simulink model "PWM_Generator"  (R2014a)
settings: Solver=ode45  StartTime=0.0  StopTime=50000  RelTol=1e-3
libraries: hdlsllib x20, simulink x5
settings Model: Creator=diloreto.m  LastModifiedBy=diloreto.m

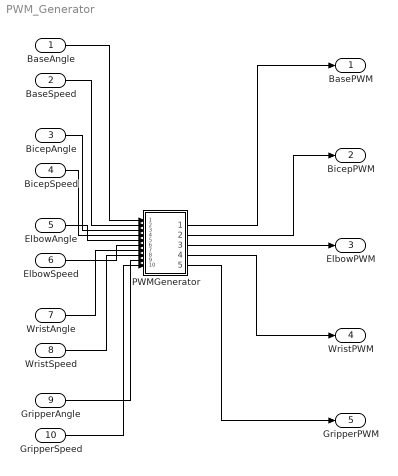
== system PWM_Generator ==
  BaseAngle : Inport  OutDataTypeStr=uint8  SampleTime=1
  BaseSpeed : Inport  Port=2  OutDataTypeStr=uint8  SampleTime=1
  BicepAngle : Inport  Port=3  OutDataTypeStr=uint8  SampleTime=1
  BicepSpeed : Inport  Port=4  OutDataTypeStr=uint8  SampleTime=1
  ElbowAngle : Inport  Port=5  OutDataTypeStr=uint8  SampleTime=1
  ElbowSpeed : Inport  Port=6  OutDataTypeStr=uint8  SampleTime=1
  WristAngle : Inport  Port=7  OutDataTypeStr=uint8  SampleTime=1
  WristSpeed : Inport  Port=8  OutDataTypeStr=uint8  SampleTime=1
  GripperAngle : Inport  Port=9  OutDataTypeStr=uint8  SampleTime=1
  GripperSpeed : Inport  Port=10  OutDataTypeStr=uint8  SampleTime=1
  PWMGenerator : Subsystem  TreatAsAtomicUnit=on  SystemSampleTime=1
  BasePWM : Outport
  BicepPWM : Outport  Port=2
  ElbowPWM : Outport  Port=3
  WristPWM : Outport  Port=4
  GripperPWM : Outport  Port=5
  wires:
  BaseAngle/1 -> PWMGenerator/1(BaseAngle)
  BaseSpeed/1 -> PWMGenerator/2(BaseSpeed)
  BicepAngle/1 -> PWMGenerator/3(BicepAngle)
  BicepSpeed/1 -> PWMGenerator/4(BicepSpeed)
  ElbowAngle/1 -> PWMGenerator/5(ElbowAngle)
  ElbowSpeed/1 -> PWMGenerator/6(ElbowSpeed)
  WristAngle/1 -> PWMGenerator/7(WristAngle)
  WristSpeed/1 -> PWMGenerator/8(WristSpeed)
  GripperAngle/1 -> PWMGenerator/9(GripperAngle)
  GripperSpeed/1 -> PWMGenerator/10(GripperSpeed)
  PWMGenerator/1(BasePWM) -> BasePWM/1
  PWMGenerator/2(BicepPWM) -> BicepPWM/1
  PWMGenerator/3(ElbowPWM) -> ElbowPWM/1
  PWMGenerator/4(WristPWM) -> WristPWM/1
  PWMGenerator/5(GripperPWM) -> GripperPWM/1

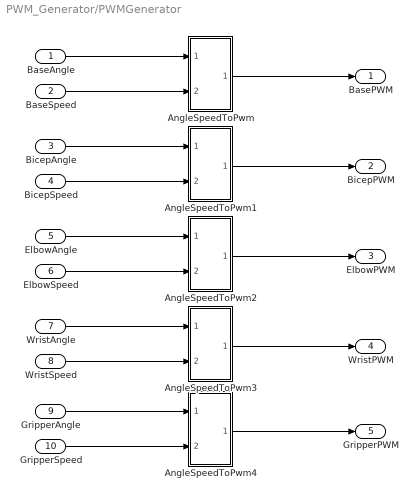
== system PWM_Generator/PWMGenerator ==
  BaseAngle : Inport  OutDataTypeStr=uint8  SampleTime=1
  BaseSpeed : Inport  Port=2  OutDataTypeStr=uint8  SampleTime=1
  BicepAngle : Inport  Port=3  OutDataTypeStr=uint8  SampleTime=1
  BicepSpeed : Inport  Port=4  OutDataTypeStr=uint8  SampleTime=1
  ElbowAngle : Inport  Port=5  OutDataTypeStr=uint8  SampleTime=1
  ElbowSpeed : Inport  Port=6  OutDataTypeStr=uint8  SampleTime=1
  WristAngle : Inport  Port=7  OutDataTypeStr=uint8  SampleTime=1
  WristSpeed : Inport  Port=8  OutDataTypeStr=uint8  SampleTime=1
  GripperAngle : Inport  Port=9  OutDataTypeStr=uint8  SampleTime=1
  GripperSpeed : Inport  Port=10  OutDataTypeStr=uint8  SampleTime=1
  AngleSpeedToPwm : Subsystem
  AngleSpeedToPwm1 : Subsystem
  AngleSpeedToPwm2 : Subsystem
  AngleSpeedToPwm3 : Subsystem
  AngleSpeedToPwm4 : Subsystem
  BasePWM : Outport
  BicepPWM : Outport  Port=2
  ElbowPWM : Outport  Port=3
  WristPWM : Outport  Port=4
  GripperPWM : Outport  Port=5
  wires:
  AngleSpeedToPwm2/1(PWM) -> ElbowPWM/1
  ElbowSpeed/1 -> AngleSpeedToPwm2/2(Speed)
  ElbowAngle/1 -> AngleSpeedToPwm2/1(Angle)
  WristAngle/1 -> AngleSpeedToPwm3/1(Angle)
  WristSpeed/1 -> AngleSpeedToPwm3/2(Speed)
  AngleSpeedToPwm3/1(PWM) -> WristPWM/1
  GripperAngle/1 -> AngleSpeedToPwm4/1(Angle)
  GripperSpeed/1 -> AngleSpeedToPwm4/2(Speed)
  AngleSpeedToPwm4/1(PWM) -> GripperPWM/1
  BaseSpeed/1 -> AngleSpeedToPwm/2(Speed)
  BaseAngle/1 -> AngleSpeedToPwm/1(Angle)
  AngleSpeedToPwm/1(PWM) -> BasePWM/1
  AngleSpeedToPwm1/1(PWM) -> BicepPWM/1
  BicepAngle/1 -> AngleSpeedToPwm1/1(Angle)
  BicepSpeed/1 -> AngleSpeedToPwm1/2(Speed)

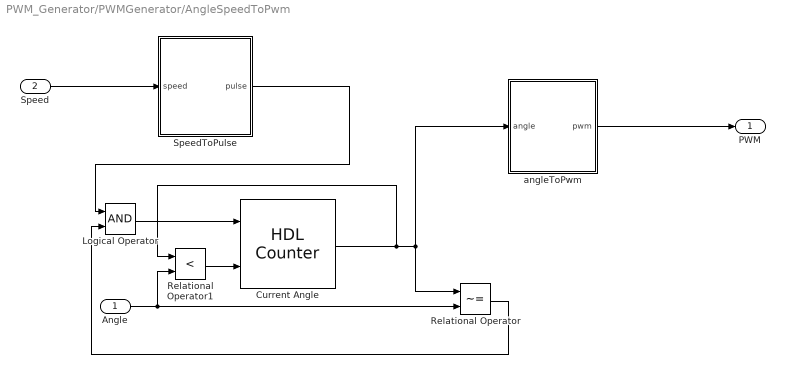
== system PWM_Generator/PWMGenerator/AngleSpeedToPwm ==
  Angle : Inport  OutDataTypeStr=uint8  SampleTime=1
  Speed : Inport  Port=2  OutDataTypeStr=uint8  SampleTime=1
  Current Angle : hdlsllib/HDL Operations/HDL Counter  CountType=Count limited  CountInit=90  CountStep=1  CountMax=180  CountFromType=Specify  CountFrom=0  CountResetPort=off  CountLoadPort=off  CountEnbPort=on  CountDirPort=on  CountDataType=Unsigned  CountWordLen=8  CountFracLen=0  CountSampTime=1
  Logical Operator : Logic  AllPortsSameDT=off  OutDataTypeStr=boolean  SampleTime=1
  Relational Operator : RelationalOperator  Operator=~=  OutDataTypeStr=boolean  SampleTime=1
  Relational Operator1 : RelationalOperator  Operator=<  OutDataTypeStr=boolean  SampleTime=1
  SpeedToPulse : Subsystem
  angleToPwm : Subsystem
  PWM : Outport  OutDataTypeStr=boolean  SampleTime=1
  wires:
  Current Angle/1 -> Relational Operator1/1, Relational Operator/1, angleToPwm/1(angle)
  Relational Operator1/1 -> Current Angle/2
  Angle/1 -> Relational Operator1/2, Relational Operator/2
  angleToPwm/1(pwm) -> PWM/1
  Speed/1 -> SpeedToPulse/1(speed)
  Logical Operator/1 -> Current Angle/1
  Relational Operator/1 -> Logical Operator/2
  SpeedToPulse/1(pulse) -> Logical Operator/1

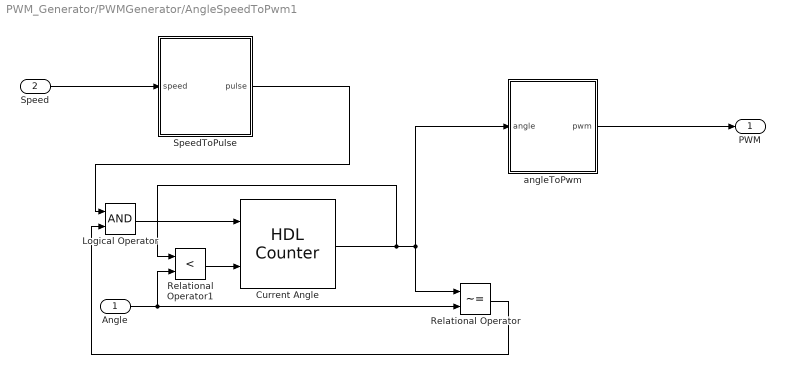
== system PWM_Generator/PWMGenerator/AngleSpeedToPwm1 ==
  Angle : Inport  OutDataTypeStr=uint8  SampleTime=1
  Speed : Inport  Port=2  OutDataTypeStr=uint8  SampleTime=1
  Current Angle : hdlsllib/HDL Operations/HDL Counter  CountType=Count limited  CountInit=90  CountStep=1  CountMax=180  CountFromType=Specify  CountFrom=0  CountResetPort=off  CountLoadPort=off  CountEnbPort=on  CountDirPort=on  CountDataType=Unsigned  CountWordLen=8  CountFracLen=0  CountSampTime=1
  Logical Operator : Logic  AllPortsSameDT=off  OutDataTypeStr=boolean  SampleTime=1
  Relational Operator : RelationalOperator  Operator=~=  OutDataTypeStr=boolean  SampleTime=1
  Relational Operator1 : RelationalOperator  Operator=<  OutDataTypeStr=boolean  SampleTime=1
  SpeedToPulse : Subsystem
  angleToPwm : Subsystem
  PWM : Outport  OutDataTypeStr=boolean  SampleTime=1
  wires:
  Current Angle/1 -> Relational Operator1/1, Relational Operator/1, angleToPwm/1(angle)
  Relational Operator1/1 -> Current Angle/2
  Angle/1 -> Relational Operator1/2, Relational Operator/2
  angleToPwm/1(pwm) -> PWM/1
  Speed/1 -> SpeedToPulse/1(speed)
  Logical Operator/1 -> Current Angle/1
  Relational Operator/1 -> Logical Operator/2
  SpeedToPulse/1(pulse) -> Logical Operator/1

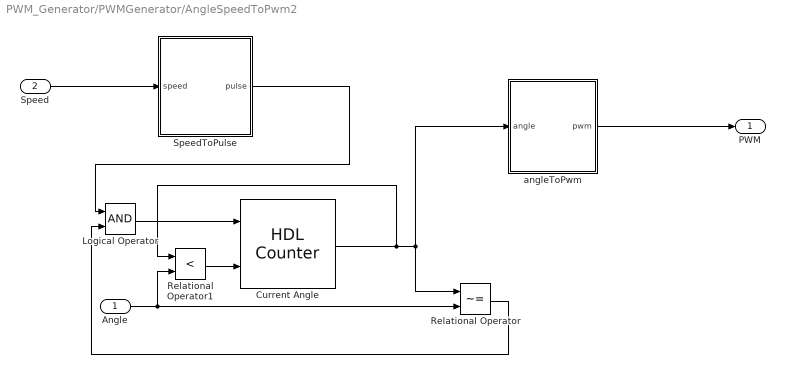
== system PWM_Generator/PWMGenerator/AngleSpeedToPwm2 ==
  Angle : Inport  OutDataTypeStr=uint8  SampleTime=1
  Speed : Inport  Port=2  OutDataTypeStr=uint8  SampleTime=1
  Current Angle : hdlsllib/HDL Operations/HDL Counter  CountType=Count limited  CountInit=90  CountStep=1  CountMax=180  CountFromType=Specify  CountFrom=0  CountResetPort=off  CountLoadPort=off  CountEnbPort=on  CountDirPort=on  CountDataType=Unsigned  CountWordLen=8  CountFracLen=0  CountSampTime=1
  Logical Operator : Logic  AllPortsSameDT=off  OutDataTypeStr=boolean  SampleTime=1
  Relational Operator : RelationalOperator  Operator=~=  OutDataTypeStr=boolean  SampleTime=1
  Relational Operator1 : RelationalOperator  Operator=<  OutDataTypeStr=boolean  SampleTime=1
  SpeedToPulse : Subsystem
  angleToPwm : Subsystem
  PWM : Outport  OutDataTypeStr=boolean  SampleTime=1
  wires:
  Current Angle/1 -> Relational Operator1/1, Relational Operator/1, angleToPwm/1(angle)
  Relational Operator1/1 -> Current Angle/2
  Angle/1 -> Relational Operator1/2, Relational Operator/2
  angleToPwm/1(pwm) -> PWM/1
  Speed/1 -> SpeedToPulse/1(speed)
  Logical Operator/1 -> Current Angle/1
  Relational Operator/1 -> Logical Operator/2
  SpeedToPulse/1(pulse) -> Logical Operator/1

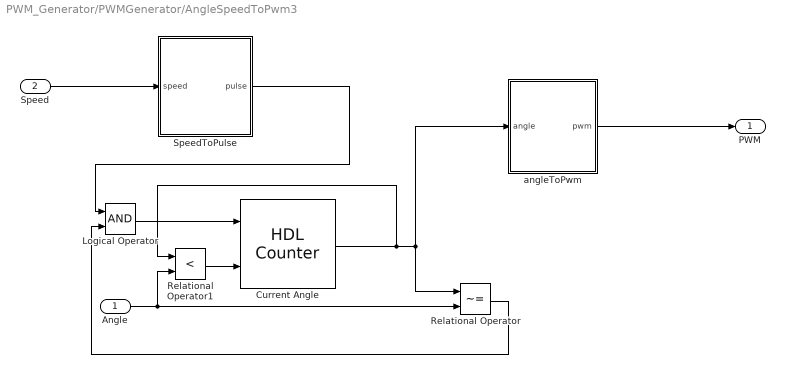
== system PWM_Generator/PWMGenerator/AngleSpeedToPwm3 ==
  Angle : Inport  OutDataTypeStr=uint8  SampleTime=1
  Speed : Inport  Port=2  OutDataTypeStr=uint8  SampleTime=1
  Current Angle : hdlsllib/HDL Operations/HDL Counter  CountType=Count limited  CountInit=90  CountStep=1  CountMax=180  CountFromType=Specify  CountFrom=0  CountResetPort=off  CountLoadPort=off  CountEnbPort=on  CountDirPort=on  CountDataType=Unsigned  CountWordLen=8  CountFracLen=0  CountSampTime=1
  Logical Operator : Logic  AllPortsSameDT=off  OutDataTypeStr=boolean  SampleTime=1
  Relational Operator : RelationalOperator  Operator=~=  OutDataTypeStr=boolean  SampleTime=1
  Relational Operator1 : RelationalOperator  Operator=<  OutDataTypeStr=boolean  SampleTime=1
  SpeedToPulse : Subsystem
  angleToPwm : Subsystem
  PWM : Outport  OutDataTypeStr=boolean  SampleTime=1
  wires:
  Current Angle/1 -> Relational Operator1/1, Relational Operator/1, angleToPwm/1(angle)
  Relational Operator1/1 -> Current Angle/2
  Angle/1 -> Relational Operator1/2, Relational Operator/2
  angleToPwm/1(pwm) -> PWM/1
  Speed/1 -> SpeedToPulse/1(speed)
  Logical Operator/1 -> Current Angle/1
  Relational Operator/1 -> Logical Operator/2
  SpeedToPulse/1(pulse) -> Logical Operator/1

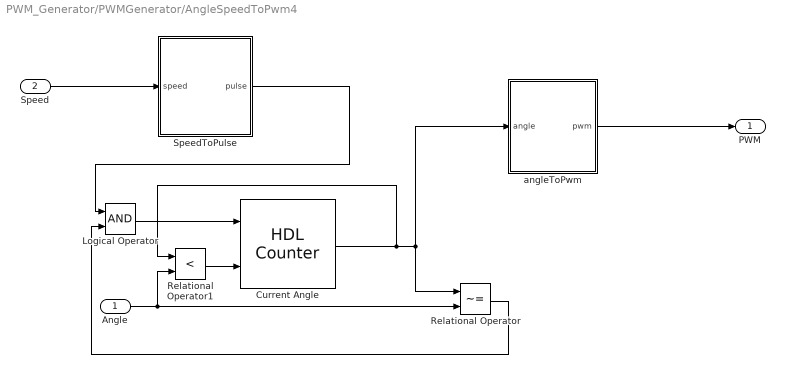
== system PWM_Generator/PWMGenerator/AngleSpeedToPwm4 ==
  Angle : Inport  OutDataTypeStr=uint8  SampleTime=1
  Speed : Inport  Port=2  OutDataTypeStr=uint8  SampleTime=1
  Current Angle : hdlsllib/HDL Operations/HDL Counter  CountType=Count limited  CountInit=90  CountStep=1  CountMax=180  CountFromType=Specify  CountFrom=0  CountResetPort=off  CountLoadPort=off  CountEnbPort=on  CountDirPort=on  CountDataType=Unsigned  CountWordLen=8  CountFracLen=0  CountSampTime=1
  Logical Operator : Logic  AllPortsSameDT=off  OutDataTypeStr=boolean  SampleTime=1
  Relational Operator : RelationalOperator  Operator=~=  OutDataTypeStr=boolean  SampleTime=1
  Relational Operator1 : RelationalOperator  Operator=<  OutDataTypeStr=boolean  SampleTime=1
  SpeedToPulse : Subsystem
  angleToPwm : Subsystem
  PWM : Outport  OutDataTypeStr=boolean  SampleTime=1
  wires:
  Current Angle/1 -> Relational Operator1/1, Relational Operator/1, angleToPwm/1(angle)
  Relational Operator1/1 -> Current Angle/2
  Angle/1 -> Relational Operator1/2, Relational Operator/2
  angleToPwm/1(pwm) -> PWM/1
  Speed/1 -> SpeedToPulse/1(speed)
  Logical Operator/1 -> Current Angle/1
  Relational Operator/1 -> Logical Operator/2
  SpeedToPulse/1(pulse) -> Logical Operator/1

== system PWM_Generator/PWMGenerator/AngleSpeedToPwm/SpeedToPulse ==
  speed : Inport  OutDataTypeStr=uint8  SampleTime=1
  Compare To Constant : simulink/Logic and Bit Operations/Compare To Constant  relop===  const=0  OutDataTypeStr=boolean
  Constant : Constant  Value=50000000  OutDataTypeStr=uint32  SampleTime=1
  Divide : Product  Inputs=*/  SampleTime=1  SaturateOnIntegerOverflow=on  RndMeth=Zero
  HDL Counter : hdlsllib/HDL Operations/HDL Counter  CountType=Count limited  CountInit=0  CountStep=1  CountMax=50000000  CountFromType=Initial value  CountFrom=0  CountResetPort=on  CountLoadPort=off  CountEnbPort=off  CountDirPort=off  CountDataType=Unsigned  CountWordLen=32  CountFracLen=0  CountSampTime=1
  Relational Operator : RelationalOperator  Operator=>  OutDataTypeStr=boolean  SampleTime=1
  pulse : Outport  SampleTime=1
  wires:
  HDL Counter/1 -> Relational Operator/1, Compare To Constant/1
  Compare To Constant/1 -> pulse/1
  Relational Operator/1 -> HDL Counter/1
  Divide/1 -> Relational Operator/2
  speed/1 -> Divide/2
  Constant/1 -> Divide/1

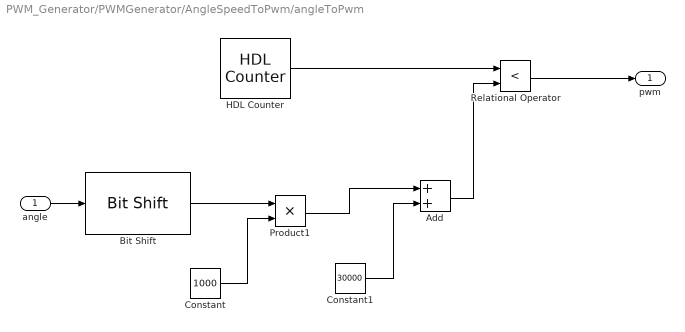
== system PWM_Generator/PWMGenerator/AngleSpeedToPwm/angleToPwm ==
  angle : Inport
  Add : Sum  OutDataTypeStr=uint32  RndMeth=Zero  SampleTime=1  SaturateOnIntegerOverflow=on
  Bit Shift : hdlsllib/HDL Operations/Bit Shift  mode=Shift Right Logical  N=1
  Constant : Constant  Value=1000  OutDataTypeStr=uint32  SampleTime=1
  Constant1 : Constant  Value=30000  OutDataTypeStr=uint32  SampleTime=1
  HDL Counter : hdlsllib/HDL Operations/HDL Counter  CountType=Count limited  CountInit=0  CountStep=1  CountMax=1000000  CountFromType=Initial value  CountFrom=0  CountResetPort=off  CountLoadPort=off  CountEnbPort=off  CountDirPort=off  CountDataType=Unsigned  CountWordLen=32  CountFracLen=0  CountSampTime=1
  Product1 : Product  OutDataTypeStr=uint32  SampleTime=1  SaturateOnIntegerOverflow=on  RndMeth=Zero
  Relational Operator : RelationalOperator  Operator=<  OutDataTypeStr=boolean  SampleTime=1
  pwm : Outport  OutDataTypeStr=boolean  SampleTime=1
  wires:
  Product1/1 -> Add/1
  angle/1 -> Bit Shift/1
  HDL Counter/1 -> Relational Operator/1
  Constant/1 -> Product1/2
  Bit Shift/1 -> Product1/1
  Add/1 -> Relational Operator/2
  Constant1/1 -> Add/2
  Relational Operator/1 -> pwm/1

== system PWM_Generator/PWMGenerator/AngleSpeedToPwm1/SpeedToPulse ==
  speed : Inport  OutDataTypeStr=uint8  SampleTime=1
  Compare To Constant : simulink/Logic and Bit Operations/Compare To Constant  relop===  const=0  OutDataTypeStr=boolean
  Constant : Constant  Value=50000000  OutDataTypeStr=uint32  SampleTime=1
  Divide : Product  Inputs=*/  SampleTime=1  SaturateOnIntegerOverflow=on  RndMeth=Zero
  HDL Counter : hdlsllib/HDL Operations/HDL Counter  CountType=Count limited  CountInit=0  CountStep=1  CountMax=50000000  CountFromType=Initial value  CountFrom=0  CountResetPort=on  CountLoadPort=off  CountEnbPort=off  CountDirPort=off  CountDataType=Unsigned  CountWordLen=32  CountFracLen=0  CountSampTime=1
  Relational Operator : RelationalOperator  Operator=>  OutDataTypeStr=boolean  SampleTime=1
  pulse : Outport  SampleTime=1
  wires:
  HDL Counter/1 -> Relational Operator/1, Compare To Constant/1
  Compare To Constant/1 -> pulse/1
  Relational Operator/1 -> HDL Counter/1
  Divide/1 -> Relational Operator/2
  speed/1 -> Divide/2
  Constant/1 -> Divide/1

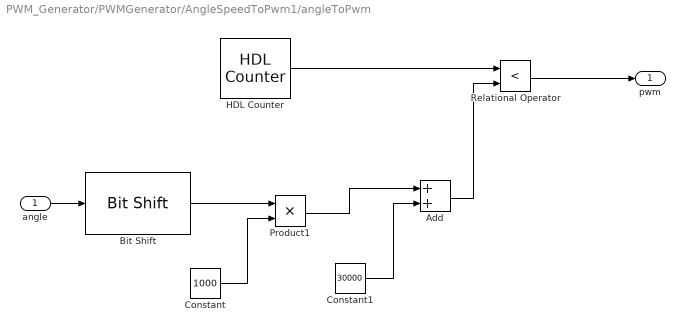
== system PWM_Generator/PWMGenerator/AngleSpeedToPwm1/angleToPwm ==
  angle : Inport
  Add : Sum  OutDataTypeStr=uint32  RndMeth=Zero  SampleTime=1  SaturateOnIntegerOverflow=on
  Bit Shift : hdlsllib/HDL Operations/Bit Shift  mode=Shift Right Logical  N=1
  Constant : Constant  Value=1000  OutDataTypeStr=uint32  SampleTime=1
  Constant1 : Constant  Value=30000  OutDataTypeStr=uint32  SampleTime=1
  HDL Counter : hdlsllib/HDL Operations/HDL Counter  CountType=Count limited  CountInit=0  CountStep=1  CountMax=1000000  CountFromType=Initial value  CountFrom=0  CountResetPort=off  CountLoadPort=off  CountEnbPort=off  CountDirPort=off  CountDataType=Unsigned  CountWordLen=32  CountFracLen=0  CountSampTime=1
  Product1 : Product  OutDataTypeStr=uint32  SampleTime=1  SaturateOnIntegerOverflow=on  RndMeth=Zero
  Relational Operator : RelationalOperator  Operator=<  OutDataTypeStr=boolean  SampleTime=1
  pwm : Outport  OutDataTypeStr=boolean  SampleTime=1
  wires:
  Product1/1 -> Add/1
  angle/1 -> Bit Shift/1
  HDL Counter/1 -> Relational Operator/1
  Constant/1 -> Product1/2
  Bit Shift/1 -> Product1/1
  Add/1 -> Relational Operator/2
  Constant1/1 -> Add/2
  Relational Operator/1 -> pwm/1

== system PWM_Generator/PWMGenerator/AngleSpeedToPwm2/SpeedToPulse ==
  speed : Inport  OutDataTypeStr=uint8  SampleTime=1
  Compare To Constant : simulink/Logic and Bit Operations/Compare To Constant  relop===  const=0  OutDataTypeStr=boolean
  Constant : Constant  Value=50000000  OutDataTypeStr=uint32  SampleTime=1
  Divide : Product  Inputs=*/  SampleTime=1  SaturateOnIntegerOverflow=on  RndMeth=Zero
  HDL Counter : hdlsllib/HDL Operations/HDL Counter  CountType=Count limited  CountInit=0  CountStep=1  CountMax=50000000  CountFromType=Initial value  CountFrom=0  CountResetPort=on  CountLoadPort=off  CountEnbPort=off  CountDirPort=off  CountDataType=Unsigned  CountWordLen=32  CountFracLen=0  CountSampTime=1
  Relational Operator : RelationalOperator  Operator=>  OutDataTypeStr=boolean  SampleTime=1
  pulse : Outport  SampleTime=1
  wires:
  HDL Counter/1 -> Relational Operator/1, Compare To Constant/1
  Compare To Constant/1 -> pulse/1
  Relational Operator/1 -> HDL Counter/1
  Divide/1 -> Relational Operator/2
  speed/1 -> Divide/2
  Constant/1 -> Divide/1

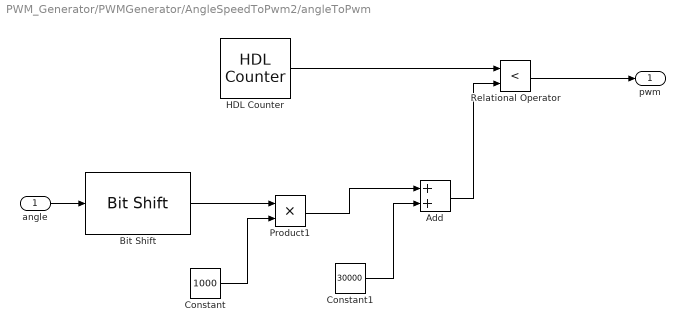
== system PWM_Generator/PWMGenerator/AngleSpeedToPwm2/angleToPwm ==
  angle : Inport
  Add : Sum  OutDataTypeStr=uint32  RndMeth=Zero  SampleTime=1  SaturateOnIntegerOverflow=on
  Bit Shift : hdlsllib/HDL Operations/Bit Shift  mode=Shift Right Logical  N=1
  Constant : Constant  Value=1000  OutDataTypeStr=uint32  SampleTime=1
  Constant1 : Constant  Value=30000  OutDataTypeStr=uint32  SampleTime=1
  HDL Counter : hdlsllib/HDL Operations/HDL Counter  CountType=Count limited  CountInit=0  CountStep=1  CountMax=1000000  CountFromType=Initial value  CountFrom=0  CountResetPort=off  CountLoadPort=off  CountEnbPort=off  CountDirPort=off  CountDataType=Unsigned  CountWordLen=32  CountFracLen=0  CountSampTime=1
  Product1 : Product  OutDataTypeStr=uint32  SampleTime=1  SaturateOnIntegerOverflow=on  RndMeth=Zero
  Relational Operator : RelationalOperator  Operator=<  OutDataTypeStr=boolean  SampleTime=1
  pwm : Outport  OutDataTypeStr=boolean  SampleTime=1
  wires:
  Product1/1 -> Add/1
  angle/1 -> Bit Shift/1
  HDL Counter/1 -> Relational Operator/1
  Constant/1 -> Product1/2
  Bit Shift/1 -> Product1/1
  Add/1 -> Relational Operator/2
  Constant1/1 -> Add/2
  Relational Operator/1 -> pwm/1

== system PWM_Generator/PWMGenerator/AngleSpeedToPwm3/SpeedToPulse ==
  speed : Inport  OutDataTypeStr=uint8  SampleTime=1
  Compare To Constant : simulink/Logic and Bit Operations/Compare To Constant  relop===  const=0  OutDataTypeStr=boolean
  Constant : Constant  Value=50000000  OutDataTypeStr=uint32  SampleTime=1
  Divide : Product  Inputs=*/  SampleTime=1  SaturateOnIntegerOverflow=on  RndMeth=Zero
  HDL Counter : hdlsllib/HDL Operations/HDL Counter  CountType=Count limited  CountInit=0  CountStep=1  CountMax=50000000  CountFromType=Initial value  CountFrom=0  CountResetPort=on  CountLoadPort=off  CountEnbPort=off  CountDirPort=off  CountDataType=Unsigned  CountWordLen=32  CountFracLen=0  CountSampTime=1
  Relational Operator : RelationalOperator  Operator=>  OutDataTypeStr=boolean  SampleTime=1
  pulse : Outport  SampleTime=1
  wires:
  HDL Counter/1 -> Relational Operator/1, Compare To Constant/1
  Compare To Constant/1 -> pulse/1
  Relational Operator/1 -> HDL Counter/1
  Divide/1 -> Relational Operator/2
  speed/1 -> Divide/2
  Constant/1 -> Divide/1

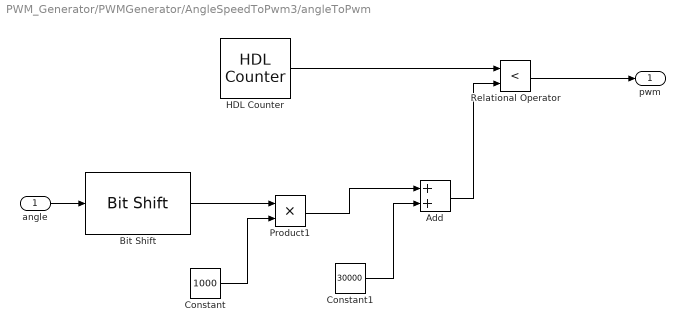
== system PWM_Generator/PWMGenerator/AngleSpeedToPwm3/angleToPwm ==
  angle : Inport
  Add : Sum  OutDataTypeStr=uint32  RndMeth=Zero  SampleTime=1  SaturateOnIntegerOverflow=on
  Bit Shift : hdlsllib/HDL Operations/Bit Shift  mode=Shift Right Logical  N=1
  Constant : Constant  Value=1000  OutDataTypeStr=uint32  SampleTime=1
  Constant1 : Constant  Value=30000  OutDataTypeStr=uint32  SampleTime=1
  HDL Counter : hdlsllib/HDL Operations/HDL Counter  CountType=Count limited  CountInit=0  CountStep=1  CountMax=1000000  CountFromType=Initial value  CountFrom=0  CountResetPort=off  CountLoadPort=off  CountEnbPort=off  CountDirPort=off  CountDataType=Unsigned  CountWordLen=32  CountFracLen=0  CountSampTime=1
  Product1 : Product  OutDataTypeStr=uint32  SampleTime=1  SaturateOnIntegerOverflow=on  RndMeth=Zero
  Relational Operator : RelationalOperator  Operator=<  OutDataTypeStr=boolean  SampleTime=1
  pwm : Outport  OutDataTypeStr=boolean  SampleTime=1
  wires:
  Product1/1 -> Add/1
  angle/1 -> Bit Shift/1
  HDL Counter/1 -> Relational Operator/1
  Constant/1 -> Product1/2
  Bit Shift/1 -> Product1/1
  Add/1 -> Relational Operator/2
  Constant1/1 -> Add/2
  Relational Operator/1 -> pwm/1

== system PWM_Generator/PWMGenerator/AngleSpeedToPwm4/SpeedToPulse ==
  speed : Inport  OutDataTypeStr=uint8  SampleTime=1
  Compare To Constant : simulink/Logic and Bit Operations/Compare To Constant  relop===  const=0  OutDataTypeStr=boolean
  Constant : Constant  Value=50000000  OutDataTypeStr=uint32  SampleTime=1
  Divide : Product  Inputs=*/  SampleTime=1  SaturateOnIntegerOverflow=on  RndMeth=Zero
  HDL Counter : hdlsllib/HDL Operations/HDL Counter  CountType=Count limited  CountInit=0  CountStep=1  CountMax=50000000  CountFromType=Initial value  CountFrom=0  CountResetPort=on  CountLoadPort=off  CountEnbPort=off  CountDirPort=off  CountDataType=Unsigned  CountWordLen=32  CountFracLen=0  CountSampTime=1
  Relational Operator : RelationalOperator  Operator=>  OutDataTypeStr=boolean  SampleTime=1
  pulse : Outport  SampleTime=1
  wires:
  HDL Counter/1 -> Relational Operator/1, Compare To Constant/1
  Compare To Constant/1 -> pulse/1
  Relational Operator/1 -> HDL Counter/1
  Divide/1 -> Relational Operator/2
  speed/1 -> Divide/2
  Constant/1 -> Divide/1

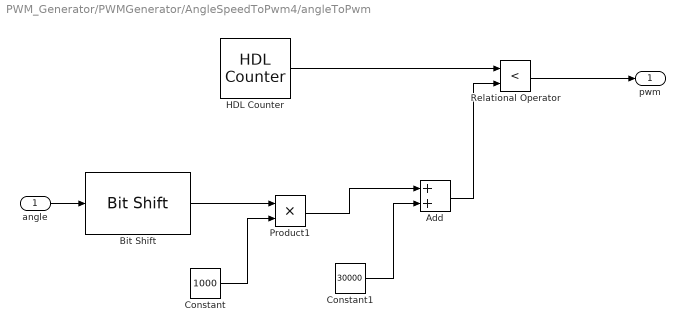
== system PWM_Generator/PWMGenerator/AngleSpeedToPwm4/angleToPwm ==
  angle : Inport
  Add : Sum  OutDataTypeStr=uint32  RndMeth=Zero  SampleTime=1  SaturateOnIntegerOverflow=on
  Bit Shift : hdlsllib/HDL Operations/Bit Shift  mode=Shift Right Logical  N=1
  Constant : Constant  Value=1000  OutDataTypeStr=uint32  SampleTime=1
  Constant1 : Constant  Value=30000  OutDataTypeStr=uint32  SampleTime=1
  HDL Counter : hdlsllib/HDL Operations/HDL Counter  CountType=Count limited  CountInit=0  CountStep=1  CountMax=1000000  CountFromType=Initial value  CountFrom=0  CountResetPort=off  CountLoadPort=off  CountEnbPort=off  CountDirPort=off  CountDataType=Unsigned  CountWordLen=32  CountFracLen=0  CountSampTime=1
  Product1 : Product  OutDataTypeStr=uint32  SampleTime=1  SaturateOnIntegerOverflow=on  RndMeth=Zero
  Relational Operator : RelationalOperator  Operator=<  OutDataTypeStr=boolean  SampleTime=1
  pwm : Outport  OutDataTypeStr=boolean  SampleTime=1
  wires:
  Product1/1 -> Add/1
  angle/1 -> Bit Shift/1
  HDL Counter/1 -> Relational Operator/1
  Constant/1 -> Product1/2
  Bit Shift/1 -> Product1/1
  Add/1 -> Relational Operator/2
  Constant1/1 -> Add/2
  Relational Operator/1 -> pwm/1
